simulink model "Magnetorquer"  (R2025b)
settings: Solver=FixedStepAuto  StartTime=0.0  StopTime=100  RelTol=1e-3
undefined symbols (not defined in the file or in its folder): juliandate, WMM2025
libraries: matrix_library x1, aerolibgravity2 x1
settings Model: Creator=chass  LastModifiedBy=chass

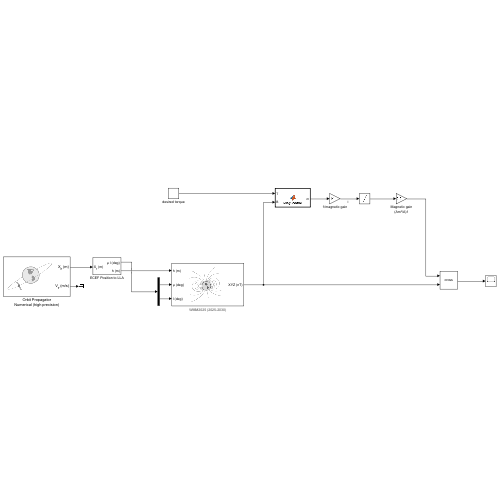
[thumbnail: Simulink's stored preview of the top-level diagram]
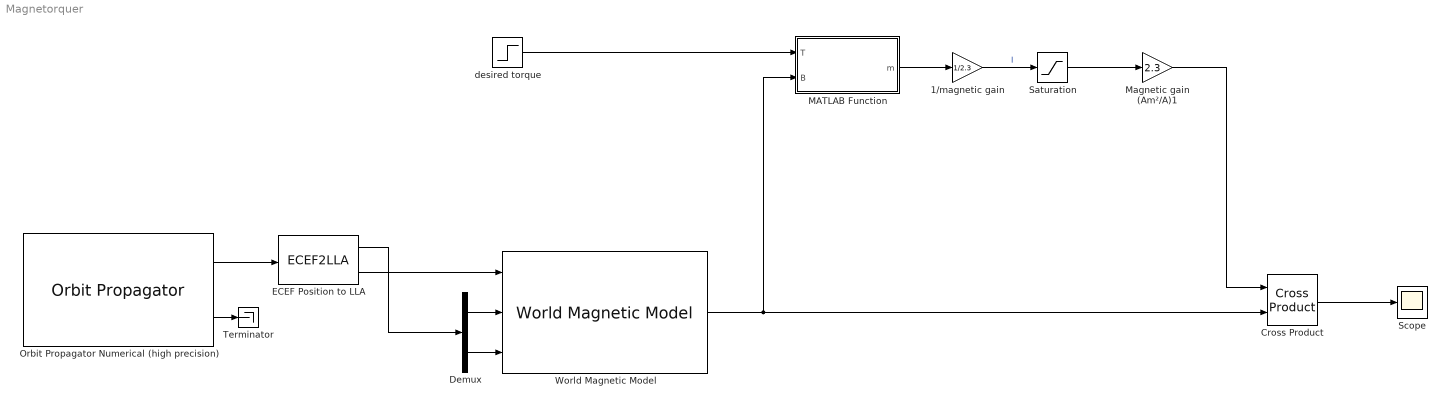
== system Magnetorquer ==
  1/magnetic gain : Gain  Gain=1/2.3
  Cross Product : matrix_library/Cross Product
  Demux : Demux  Outputs=2
  ECEF Position to LLA : ECEF2LLA
  MATLAB Function : MATLAB Function  TreatAsAtomicUnit=on
  Magnetic gain (Am²/A)1 : Gain  Gain=2.3
  Orbit Propagator Numerical (high precision) : OrbitPropagator  propagator=Numerical (high precision)  outportFrame=Fixed-frame  startDate=juliandate(2025, 1, 1, 12, 0, 0)  dateOut=off  inertialPosition=[3649700.0 3308200.0 -4676600.0]  inertialVelocity=[-2750.8 6666.4 2573.4]  fixedPosition=[-4142689.0 -2676864.7 -4669861.6]  fixedVelocity=[1452.7 -6720.7 2568.1]  customR=3396200  customMu=4.305e13  customJ2=1.0826269e-03  customOmega=4.06125949e-3
  Saturation : Saturate  UpperLimit=84e-3  LowerLimit=-84e-3
  Scope : Scope
      settings: ActiveDisplayYMinimum=-1.9768714932853444  ActiveDisplayYMaximum=14.85447556721385
  Terminator : Terminator
  World Magnetic Model : aerolibgravity2/World Magnetic Model  model=WMM2025 (2025-2030)  customFile='WMM2025.COF'  units=Metric (MKS)  time_in=off  month=January  day=1  year=2025  action=Error  h_out=off  dec_out=off  inc_out=off  ti_out=off
  desired torque : Step  SampleTime=0
  wires:
  Cross Product/1 -> Scope/1
  Orbit Propagator Numerical (high precision)/2 -> Terminator/1
  Orbit Propagator Numerical (high precision)/1 -> ECEF Position to LLA/1
  ECEF Position to LLA/1 -> Demux/1
  World Magnetic Model/1 -> Cross Product/2, MATLAB Function/2(B)
  Demux/1 -> World Magnetic Model/2
  Demux/2 -> World Magnetic Model/3
  ECEF Position to LLA/2 -> World Magnetic Model/1
  desired torque/1 -> MATLAB Function/1(T)
  MATLAB Function/1(m) -> 1/magnetic gain/1
  1/magnetic gain/1 -> Saturation/1  "I"
  Saturation/1 -> Magnetic gain (Am²/A)1/1
  Magnetic gain (Am²/A)1/1 -> Cross Product/1

== matlab function Magnetorquer/MATLAB Function ==
  data: T input; B input; m output
function m = MagControl(T, B)

m = 1/(norm(B)^2) * cross(T, -B);
